simulink model "USCity"  (R2024b)
settings: Solver=FixedStepAuto  StartTime=0.0  StopTime=Ts  FixedStep=0.001  RelTol=1e-3
PreLoadFcn:
  | setUpUSCity
model workspace (MAT data in the model file):
  firstWarning = 0
  originalScenarioChecksum = 'F73A6DA3C723D3CA73A6F931B7A52A9C'
values from neighbouring files (symbols this model uses):
  C = [0;temp2/m - v;0;temp3]    [LQR_Coeff_US_city.m]
  K = lqr(A,B,Q,R)    [LQR_Coeff_US_city.m]
  m = 2000    [LQR_Coeff_US_city.m]
  psi_o = 0    [setUpUSCity.m]
  s = size(xRef)    [setUpUSCity.m]
  vel = lookUpt(2:27,2:32)    [setUpUSCity.m]
  X_o = refPose(1,1)    [setUpUSCity.m]
  xlt = lookUpt(2:27,1)    [setUpUSCity.m]
  xRef = refPose(:,1)    [setUpUSCity.m]
  Y_o = -refPose(1,2)    [setUpUSCity.m]
  ylt = lookUpt(1,2:32)    [setUpUSCity.m]
  yRef = -refPose(:,2)    [setUpUSCity.m]
undefined symbols (not defined in the file or in its folder): deg, DiscIntNeverNeededParam, rad
libraries: simulink x12, slpidlib x4, autolibutils x4, autolibshared x3, vehdynlibviscommon x1, aerolibconvert2 x1, simulink_extras x1, drivingscenarioandsensors x1, sim3dlib x1, sim3dautolib x1
(part 3 of 3)

== system USCity/Lateral and Longitudinal Controller/Controller/LPF2 ==
  u : Inport
  k : Inport  Port=2
  Add1 : Sum
  Product : Product
  Subtract : Sum  Inputs=+-
  Unit Delay : UnitDelay  SampleTime=-1  HasFrameUpgradeWarning=on
  y : Outport
  wires:
  k/1 -> Product/1
  Product/1 -> Add1/1
  Add1/1 -> y/1, Unit Delay/1
  Unit Delay/1 -> Subtract/2, Add1/2
  u/1 -> Subtract/1
  Subtract/1 -> Product/2

== system USCity/Lateral and Longitudinal Controller/Controller/LPF3 ==
  u : Inport
  k : Inport  Port=2
  Add1 : Sum
  Product : Product
  Subtract : Sum  Inputs=+-
  Unit Delay : UnitDelay  SampleTime=-1  HasFrameUpgradeWarning=on
  y : Outport
  wires:
  k/1 -> Product/1
  Product/1 -> Add1/1
  Add1/1 -> y/1, Unit Delay/1
  Unit Delay/1 -> Subtract/2, Add1/2
  u/1 -> Subtract/1
  Subtract/1 -> Product/2

== system USCity/Lateral and Longitudinal Controller/Controller/LPF4 ==
  u : Inport
  k : Inport  Port=2
  Add1 : Sum
  Product : Product
  Subtract : Sum  Inputs=+-
  Unit Delay : UnitDelay  SampleTime=-1  HasFrameUpgradeWarning=on
  y : Outport
  wires:
  k/1 -> Product/1
  Product/1 -> Add1/1
  Add1/1 -> y/1, Unit Delay/1
  Unit Delay/1 -> Subtract/2, Add1/2
  u/1 -> Subtract/1
  Subtract/1 -> Product/2

== system USCity/Lateral and Longitudinal Controller/Controller/LPF5 ==
  u : Inport
  k : Inport  Port=2
  Add1 : Sum
  Product : Product
  Subtract : Sum  Inputs=+-
  Unit Delay : UnitDelay  SampleTime=-1  HasFrameUpgradeWarning=on
  y : Outport
  wires:
  k/1 -> Product/1
  Product/1 -> Add1/1
  Add1/1 -> y/1, Unit Delay/1
  Unit Delay/1 -> Subtract/2, Add1/2
  u/1 -> Subtract/1
  Subtract/1 -> Product/2

== system USCity/Lateral and Longitudinal Controller/Controller/LPF6 ==
  u : Inport
  k : Inport  Port=2
  Add1 : Sum
  Product : Product
  Subtract : Sum  Inputs=+-
  Unit Delay : UnitDelay  SampleTime=-1  HasFrameUpgradeWarning=on
  y : Outport
  wires:
  k/1 -> Product/1
  Product/1 -> Add1/1
  Add1/1 -> y/1, Unit Delay/1
  Unit Delay/1 -> Subtract/2, Add1/2
  u/1 -> Subtract/1
  Subtract/1 -> Product/2

== system USCity/Lateral and Longitudinal Controller/Controller/LPF7 ==
  u : Inport
  k : Inport  Port=2
  Add1 : Sum
  Product : Product
  Subtract : Sum  Inputs=+-
  Unit Delay : UnitDelay  SampleTime=-1  HasFrameUpgradeWarning=on
  y : Outport
  wires:
  k/1 -> Product/1
  Product/1 -> Add1/1
  Add1/1 -> y/1, Unit Delay/1
  Unit Delay/1 -> Subtract/2, Add1/2
  u/1 -> Subtract/1
  Subtract/1 -> Product/2

== system USCity/Lateral and Longitudinal Controller/Controller2/LPF ==
  u : Inport
  k : Inport  Port=2
  Add1 : Sum
  Product : Product
  Subtract : Sum  Inputs=+-
  Unit Delay : UnitDelay  SampleTime=-1  HasFrameUpgradeWarning=on
  y : Outport
  wires:
  k/1 -> Product/1
  Product/1 -> Add1/1
  Add1/1 -> y/1, Unit Delay/1
  Unit Delay/1 -> Subtract/2, Add1/2
  u/1 -> Subtract/1
  Subtract/1 -> Product/2

== system USCity/Lateral and Longitudinal Controller/Controller2/LPF1 ==
  u : Inport
  k : Inport  Port=2
  Add1 : Sum
  Product : Product
  Subtract : Sum  Inputs=+-
  Unit Delay : UnitDelay  SampleTime=-1  HasFrameUpgradeWarning=on
  y : Outport
  wires:
  k/1 -> Product/1
  Product/1 -> Add1/1
  Add1/1 -> y/1, Unit Delay/1
  Unit Delay/1 -> Subtract/2, Add1/2
  u/1 -> Subtract/1
  Subtract/1 -> Product/2

== system USCity/Lateral and Longitudinal Controller/Controller2/LPF2 ==
  u : Inport
  k : Inport  Port=2
  Add1 : Sum
  Product : Product
  Subtract : Sum  Inputs=+-
  Unit Delay : UnitDelay  SampleTime=-1  HasFrameUpgradeWarning=on
  y : Outport
  wires:
  k/1 -> Product/1
  Product/1 -> Add1/1
  Add1/1 -> y/1, Unit Delay/1
  Unit Delay/1 -> Subtract/2, Add1/2
  u/1 -> Subtract/1
  Subtract/1 -> Product/2

== system USCity/Powertrain & Driveline/Driveline/AWD ==
  TPowertrain : Inport
  AWD : Gain  Gain=[1;1;1;1]./2
  TAxles : Outport  VectorParamsAs1DForOutWhenUnconnected=off
  wires:
  TPowertrain/1 -> AWD/1
  AWD/1 -> TAxles/1

== system USCity/Powertrain & Driveline/Driveline/FWD ==
  TPowertrain : Inport
  FWD : Gain  Gain=[1;1;0;0]
  TAxles : Outport  VectorParamsAs1DForOutWhenUnconnected=off
  wires:
  FWD/1 -> TAxles/1
  TPowertrain/1 -> FWD/1

== system USCity/Powertrain & Driveline/Driveline/RWD ==
  TPowertrain : Inport
  RWD : Gain  Gain=[0;0;1;1]
  TAxles : Outport  VectorParamsAs1DForOutWhenUnconnected=off
  wires:
  TPowertrain/1 -> RWD/1
  RWD/1 -> TAxles/1

== matlab function USCity/Lateral and Longitudinal Controller/Controller/MATLAB Function ==
  data: pose input; e output; way_point input; v input; cte output; yaw_ref output; yaw output; y output
function [e,cte,yaw_ref,yaw,y]= error(pose,way_point,v)

    x = pose(1);
    y = pose(2);
    yaw = pose(3);

    nearest_idx = find_nearest_waypoint(x,y,way_point);
    [cte,heading_error,yaw_ref]= compute_cte(x,y,yaw,way_point,nearest_idx,v);    



e = heading_error;
end


function idx = find_nearest_waypoint(x, y, waypoints)
    dists = vecnorm((waypoints - [x, y]).');
    [~, idx] = min(dists);
end
 
function [cte,heading_error,yaw_ref] = compute_cte(x,y,yaw,way_point,idx,v)
    wp1 = way_point(idx,:);
    wp1 = wp1';

    if idx < size(way_point,1)
        wp2 = way_point(idx+1,:);
    else
        wp2 = wp1;
    end
    wp2 = wp2';


    dx = wp2(1) - wp1(1);
    dy = wp2(2) - wp1(2);

    target_angle = atan2(dy, dx);
    heading_error = target_angle - yaw;

    cte = -sin(yaw) * dx + cos(yaw) * dy;
    cte = v*sin(yaw + heading_error);

    

    seg_vec = [dx,dy];
    pos_vec = [x-wp1(1),y-wp1(2)];
    cross_val = dx * pos_vec(2) - dy * pos_vec(1);
    seg_len = norm(seg_vec) + 1e-6;
    cte = (cross_val / seg_len);
    heading_error = rem(heading_error+pi,2*pi) - pi;
    yaw_ref = target_angle;


    
end

== matlab function USCity/Lateral and Longitudinal Controller/Controller/MATLAB Function1 ==
  data: cte input; heading_error input; v input; pose input; u output; heading_error_rate input; yawrate_ref input; cte_dot input; K input
function u = lqr(cte,heading_error,v,pose,heading_error_rate,yawrate_ref,cte_dot,K)

    x = pose(1);
    y = pose(2);
    yaw = pose(3);
    Iz = 4000; %kg*m^2
    la = 1.4; %m
    lb = 1.6; %4
    h = 0.35; %m
    m = 2000; %m
    tw = 1.4; %m
    Cf = 2*12000; % N/rad
    Cr = 2*11000; %N/rad


    
    % cte_dot = v*cos(yaw)*heading_error + v*sin(yaw);
    e_vec = [cte,cte_dot,heading_error,heading_error_rate]';
    
    u = (K(3)*e_vec(3)+K(4)*e_vec(4))+0.001*yawrate_ref*(la+lb)/10;
 


    

end

== matlab function USCity/Lateral and Longitudinal Controller/Controller/MATLAB Function2 ==
  data: cte input; heading_error input; v input; pose input; u output; heading_error_rate input; yawrate_ref input; cte_dot input; K1 input; K2 input
function u = smc(cte,heading_error,v,pose,heading_error_rate,yawrate_ref,cte_dot,K1,K2)

    x = pose(1);
    y = pose(2);
    yaw = pose(3);
    Iz = 4000; %kg*m^2
    la = 1.4; %m
    lb = 1.6; %4
    h = 0.35; %m
    m = 2000; %m
    tw = 1.4; %m
    Cf = 2*12000; % N/rad
    Cr = 2*11000; %N/rad
    v = 10;
    temp2 = -(Cf + Cr)/m;
    temp1 = -(Cf*la - Cr*lb);
    temp3 = -(Cf*la^2 + Cr*lb^2)/v/Iz;

    
    cte_dot = v*cos(yaw)*heading_error + v*sin(yaw);
    e_vec = [cte,cte_dot,heading_error,heading_error_rate]';

    c1 = 0.071;
    c2 = 0.05;
    c3 = -0.07;
    c4 = -0.3;

    s = c1*cte_dot + c2*heading_error + c3*heading_error_rate + c4*cte;
    
    u = -m*(-(temp1/m/v - v)*yawrate_ref - temp2*cte_dot/v + temp2*heading_error - temp2*(heading_error_rate)/m/v - K1 *tanh(s) - c2*heading_error_rate/c1 - K2*s )/Cf;

    

end

== matlab function USCity/Lateral and Longitudinal Controller/Controller/MATLAB Function3 ==
  data: cte input; heading_error input; v input; pose input; u output; heading_error_rate_mrac output; heading_error_rate input; yawrate_ref input; cte_dot input; yaw_rate input; y_dot input; heading_error_rate_mrac_prev input; cte_dot_mrac_prev input; theta_hat_prev input; theta_hat_prev1 input; gamma input; theta_hat output; theta1_hat output; cte_dot_mrac output
function [u,heading_error_rate_mrac,theta_hat,theta1_hat,cte_dot_mrac]= mrac(cte,heading_error,v,pose,heading_error_rate,yawrate_ref,cte_dot,yaw_rate,y_dot,heading_error_rate_mrac_prev,cte_dot_mrac_prev,theta_hat_prev,theta_hat_prev1,gamma)


    x = pose(1);
    y = pose(2);
    yaw = pose(3);
    
    Iz = 4000; %kg*m^2
    la = 1.4; %m
    lb = 1.6; %4
    h = 0.35; %m
    m = 2000; %m
    tw = 1.4; %m
    Cf = 2*12000; % N/rad
    Cr = 2*11000; %N/rad
    dt = 0.001;

    % 


    c2 = (Cf*la - Cr*lb)/Iz;
    c1 = -c2/v;
    c3 = -(Cf*la^2 + Cr*lb^2)/Iz/v;
    c4 = -(Cf +Cr)/m;
    c5 = -v - (Cf*la - Cr*lb)/m/v;
    c6 = -(Cf*la - Cr*lb)/m/v;
    am = -10000;
    am1 = -100;

    k = -0.03;



    heading_error_rate_mrac_dot = am*heading_error_rate_mrac_prev;

    heading_error_rate_mrac = heading_error_rate_mrac_prev + heading_error_rate_mrac_dot*dt;
    cte_ddot = am1*cte_dot_mrac_prev;
    cte_dot_mrac = cte_dot_mrac_prev + cte_ddot*dt;


    u = -(theta_hat_prev*heading_error_rate_mrac + theta_hat_prev1*cte_dot_mrac + c1*cte_dot + c2*heading_error + c3*heading_error_rate + c3*yawrate_ref) + k*cte;

    e = heading_error_rate;

    theta_dot =  -gamma * e * heading_error_rate;
    theta_hat = theta_hat_prev + dt*theta_dot;

    theta1_dot =  -gamma * cte_dot * cte_dot;
    theta1_hat = theta_hat_prev1 + dt*theta1_dot;




end

== matlab function USCity/Lateral and Longitudinal Controller/Controller2/MATLAB Function ==
  data: pose input; e output; way_point input; v input; cte output; yaw_ref output
function [e,cte,yaw_ref]= error(pose,way_point,v)

    x = pose(1);
    y = pose(2);
    yaw = pose(3);

    nearest_idx = find_nearest_waypoint(x,y,way_point);
    [cte,heading_error,yaw_ref]= compute_cte(x,y,yaw,way_point,nearest_idx,v);    



e = heading_error;
end


function idx = find_nearest_waypoint(x, y, waypoints)
    dists = vecnorm((waypoints - [x, y]).');
    [~, idx] = min(dists);
end
 
function [cte,heading_error,yaw_ref] = compute_cte(x,y,yaw,way_point,idx,v)
    wp1 = way_point(idx,:);
    wp1 = wp1';

    if idx < size(way_point,1)
        wp2 = way_point(idx+1,:);
    else
        wp2 = wp1;
    end
    wp2 = wp2';


    dx = wp2(1) - wp1(1);
    dy = wp2(2) - wp1(2);

    target_angle = atan2(dy, dx);
    heading_error = target_angle - yaw;
    % if heading_error > pi
    %     heading_error = heading_error - 2 * pi;
    % elseif heading_error < -pi
    %     heading_error = heading_error + 2 * pi;
    % end
     

    cte = -sin(yaw) * dx + cos(yaw) * dy;
    cte = v*sin(yaw + heading_error);

    

    seg_vec = [dx,dy];
    pos_vec = [x-wp1(1),y-wp1(2)];
    cross_val = dx * pos_vec(2) - dy * pos_vec(1);
    seg_len = norm(seg_vec) + 1e-6;
    cte = (cross_val / seg_len);
    heading_error = rem(heading_error+pi,2*pi) - pi;
    yaw_ref = target_angle;


    
end

== matlab function USCity/Final Trajectory Bird's-Eye Visualization/MATLAB Function ==
  data: pos input; egoActor output Bus: BusActorsActors; vel input; yaw input; yawRate input
function egoActor = packEgo(pos,vel,yaw,yawRate)
% Pack ego information into a single ego actor bus
%
% Imoprtant note:
% Output is a bus of type BusActorsActors. This is the same bus used by the
% Scenario Reader to output an individual actor. If you change the
% output bus name of Scenario Reader, change the output bus name here
% as well by clicking on 'Edit Data' in the menu above.

egoActor = struct(...
    'ActorID',67,...
    'Position', [pos(1) pos(2) 0], ...
    'Velocity', [vel(1) vel(2) 0], ...
    'Roll', 0, ...
    'Pitch', 0, ...
    'Yaw', yaw, ...
    'AngularVelocity', [0 0 yawRate]);

== matlab function USCity/Lateral and Longitudinal Controller/Controller2/MATLAB Function1 ==
  data: cte input; heading_error input; v input; pose input; u output; heading_error_rate input; yawrate_ref input; K input
function u = lqr(cte,heading_error,v,pose,heading_error_rate,yawrate_ref,K)

    x = pose(1);
    y = pose(2);
    yaw = pose(3);
    Iz = 4000; %kg*m^2
    la = 1.4; %m
    lb = 1.6; %4
    h = 0.35; %m
    m = 2000; %m
    tw = 1.4; %m
    Cf = 2*12000; % N/rad
    Cr = 2*11000; %N/rad
    v = 10;

    
    cte_dot = v*cos(yaw)*heading_error + v*sin(yaw);
    e_vec = [cte,cte_dot,heading_error,heading_error_rate]';
    
    u = (K(1)*e_vec(1)+K(2)*e_vec(2)+K(3)*e_vec(3)+K(4)*e_vec(4))+heading_error+0.001*yawrate_ref*(la+lb)/10;

 


    

end

== matlab function USCity/Lateral and Longitudinal Controller/Controller2/MATLAB Function2 ==
  data: cte input; heading_error input; v input; pose input; u output; heading_error_rate input; yawrate_ref input; cte_dot input; cte_int input; K1 input; K2 input
function u = smc(cte,heading_error,v,pose,heading_error_rate,yawrate_ref,cte_dot,cte_int,K1,K2)

    x = pose(1);
    y = pose(2);
    yaw = pose(3);
    Iz = 4000; %kg*m^2
    la = 1.4; %m
    lb = 1.6; %4
    h = 0.35; %m
    m = 2000; %m
    tw = 1.4; %m
    Cf = 2*12000; % N/rad
    Cr = 2*11000; %N/rad
    v = 10;
    temp2 = -(Cf + Cr)/m;
    temp1 = -(Cf*la - Cr*lb);
    temp3 = -(Cf*la^2 + Cr*lb^2)/v/Iz;



    
    cte_dot = v*cos(yaw)*heading_error + v*sin(yaw);
    
    e_vec = [cte,cte_dot,heading_error,heading_error_rate]';

    c1 = 0.0028;
    c2 = 0.05;
    c3 = -0.01;

    s = c1*cte_dot + c2*heading_error + c3*cte_int; 
    
    u = -m*(-(temp1/m/v - v)*yawrate_ref - temp2*cte_dot/v + temp2*heading_error - temp2*(heading_error_rate)/m/v - K1 *tanh(s) - c2*heading_error_rate/c1 - K2*s )/Cf;

    

end

== matlab function USCity/Lateral and Longitudinal Controller/Controller2/MATLAB Function3 ==
  data: cte input; heading_error input; v input; pose input; u output; heading_error_rate input; yawrate_ref input; cte_dot input; k1 input; k2 input; error_selection input
function u  = mrac(cte,heading_error,v,pose,heading_error_rate,yawrate_ref,cte_dot,k1,k2,error_selection)


    x = pose(1);
    y = pose(2);
    yaw = pose(3);
    
    Iz = 4000; %kg*m^2
    la = 1.4; %m
    lb = 1.6; %4
    h = 0.35; %m
    m = 2000; %m
    tw = 1.4; %m
    Cf = 2*12000; % N/rad
    Cr = 2*11000; %N/rad

    % 


    if error_selection == 1

        c2 = -(Cf + Cr)/(m*v);
        c1 = -(la*Cf - lb*Cr)/v/m - v;
        c3 = -c2 ;
        c4 = c1 + v;
        u = m*(k1*cte_dot + c1*yawrate_ref + c2*cte_dot + c3*heading_error + c4*heading_error_rate)/Cf;
    else if error_selection == 2

        c2 = (Cf*la - Cr*lb)/Iz;
        c1 = -c2/v;
        c3 = -(Cf*la^2 + Cr*lb^2)/Iz/v;
    
        u = -m*(k2*heading_error_rate + c1*cte_dot + c2*heading_error + c3*heading_error_rate + c3*yawrate_ref)/Cf;
    else
        u = 0;
    end










end
